simulink model "Cascade"  (R2020b)
settings: Solver=VariableStepAuto  StartTime=0.0  StopTime=10.0  RelTol=1e-3
settings Model: Creator=Akshata Ashok  LastModifiedBy=Akshata Ashok

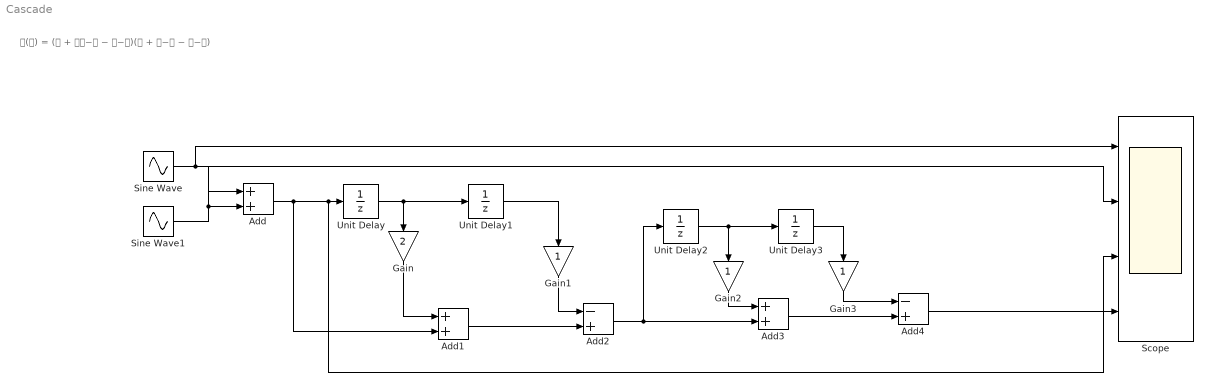
== system Cascade ==
  note: 𝐇(𝐳) = (𝟏 + 𝟐𝐳−𝟏 − 𝐳−𝟐)(𝟏 + 𝐳−𝟏 − 𝐳−𝟐)
  Add : Sum
  Add1 : Sum
  Add2 : Sum  Inputs=-+
  Add3 : Sum
  Add4 : Sum  Inputs=-+
  Gain : Gain  Gain=2
  Gain1 : Gain
  Gain2 : Gain
  Gain3 : Gain
  Scope : Scope  NumInputPorts=4
  Sine Wave : Sin  Frequency=10  SampleTime=0
  Sine Wave1 : Sin  Frequency=50  SampleTime=0
  Unit Delay{,1..3} (4 alike) : UnitDelay  SampleTime=-1  HasFrameUpgradeWarning=on
  wires:
  Sine Wave/1 -> Scope/1, Add/1
  Sine Wave1/1 -> Add/2, Scope/2
  Add/1 -> Add1/2, Scope/3, Unit Delay/1
  Unit Delay/1 -> Gain/1, Unit Delay1/1
  Gain/1 -> Add1/1
  Unit Delay1/1 -> Gain1/1
  Gain1/1 -> Add2/1
  Add1/1 -> Add2/2
  Add2/1 -> Unit Delay2/1, Add3/2
  Unit Delay2/1 -> Gain2/1, Unit Delay3/1
  Gain2/1 -> Add3/1
  Unit Delay3/1 -> Gain3/1
  Gain3/1 -> Add4/1
  Add3/1 -> Add4/2
  Add4/1 -> Scope/4
